simulink model "linear_controller_linear_plant_mks_sim"  (R2022b)
settings: Solver=VariableStepAuto  StartTime=0.0  StopTime=4500  FixedStep=0.5  RelTol=1e-6
undefined symbols (not defined in the file): u0, x0
libraries: mpclib x1
settings Model: Creator=Mitarbeiter  LastModifiedBy=Mitarbeiter

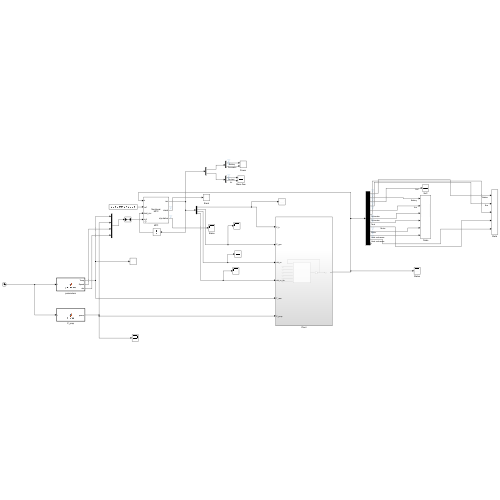
[thumbnail: Simulink's stored preview of the top-level diagram]
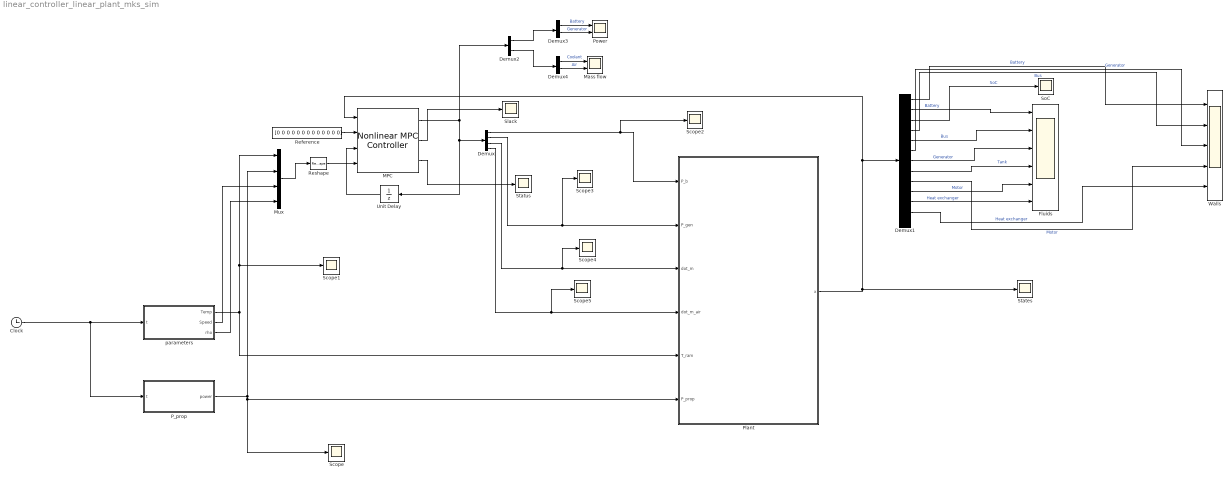
== system linear_controller_linear_plant_mks_sim ==
  Clock : Clock
  Demux : Demux
  Demux1 : Demux  Outputs=13
  Demux2 : Demux  Outputs=2
  Demux3 : Demux  Outputs=2
  Demux4 : Demux  Outputs=2
  Fluids : Scope  NumInputPorts=6
  MPC : mpclib/Nonlinear MPC Controller  nlmpcobj=nlobj  UseObjectTs=on  UseMEX=off  md_enabled=on  mvtarget_enabled=off  param_enabled=off  cost_enabled=off  mvseq_enabled=off  stateseq_enabled=off  ovseq_enabled=off  slack_enabled=on  status_enabled=on  ov_min=off  ov_max=off  mv_min=off  mv_max=off  mvrate_min=off  mvrate_max=off  state_min=off  state_max=off  ov_weight=off  mv_weight=off  mvrate_weight=off  ecr_weight=off  nlp_initialize=off
  Mass flow : Scope  NumInputPorts=2
  Mux : Mux
  P_prop : MATLAB Function  TreatAsAtomicUnit=on
  Plant : Subsystem
  Power : Scope  NumInputPorts=2
  Reference : Constant  Value=[0 0 0 0 0 0 0 0 0 0 0 0 0]  VectorParams1D=off
  Reshape : Reshape  OutputDimensionality=Row vector (2-D)
  Scope{,1..5} (6 alike) : Scope
  Slack : Scope
  SoC : Scope
  States : Scope
  Status : Scope
  Unit Delay : UnitDelay  InitialCondition=u0  SampleTime=-1  HasFrameUpgradeWarning=on
  Walls : Scope  NumInputPorts=5
  parameters : MATLAB Function  TreatAsAtomicUnit=on
  wires:
  Clock/1 -> parameters/1(t), P_prop/1(t)
  parameters/1(Temp) -> Scope1/1, Mux/1, Plant/5(T_ram)
  P_prop/1(power) -> Scope/1, Plant/6(P_prop), Mux/2
  Plant/1(x) -> MPC/1, Demux1/1, States/1
  Reference/1 -> MPC/2
  Demux/1 -> Scope2/1, Plant/1(P_b)
  Demux/2 -> Scope3/1, Plant/2(P_gen)
  MPC/1 -> Demux2/1, Demux/1, Unit Delay/1
  Mux/1 -> Reshape/1
  Unit Delay/1 -> MPC/3
  Reshape/1 -> MPC/4
  Demux1/3 -> SoC/1  "SoC"
  MPC/3 -> Status/1
  Demux/3 -> Scope4/1, Plant/3(dot_m)
  Demux/4 -> Scope5/1, Plant/4(dot_m_air)
  parameters/2(Speed) -> Mux/3
  MPC/2 -> Slack/1
  parameters/3(rho) -> Mux/4
  Demux4/1 -> Mass flow/1  "Coolant"
  Demux4/2 -> Mass flow/2  "Air"
  Demux3/2 -> Power/2  "Generator"
  Demux3/1 -> Power/1  "Battery"
  Demux2/1 -> Demux3/1
  Demux2/2 -> Demux4/1
  Demux1/1 -> Walls/1  "Battery"
  Demux1/2 -> Fluids/1  "Battery"
  Demux1/4 -> Walls/2  "Bus"
  Demux1/5 -> Fluids/2  "Bus"
  Demux1/6 -> Walls/3  "Generator"
  Demux1/7 -> Fluids/3  "Generator"
  Demux1/8 -> Fluids/4  "Tank"
  Demux1/9 -> Walls/4  "Motor"
  Demux1/10 -> Fluids/5  "Motor"
  Demux1/11 -> Fluids/6  "Heat exchanger"
  Demux1/12 -> Walls/5  "Heat exchanger"

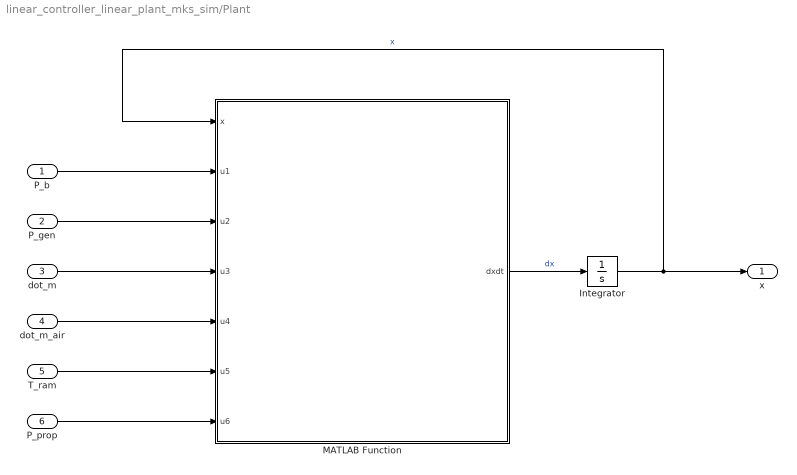
== system linear_controller_linear_plant_mks_sim/Plant ==
  P_b : Inport
  P_gen : Inport  Port=2
  dot_m : Inport  Port=3
  dot_m_air : Inport  Port=4
  T_ram : Inport  Port=5
  P_prop : Inport  Port=6
  Integrator : Integrator  InitialCondition=x0
  MATLAB Function : MATLAB Function  TreatAsAtomicUnit=on
  x : Outport
  wires:
  MATLAB Function/1(dxdt) -> Integrator/1  "dx"
  Integrator/1 -> x/1, MATLAB Function/1(x)  "x"
  P_prop/1 -> MATLAB Function/7(u6)
  P_b/1 -> MATLAB Function/2(u1)
  dot_m/1 -> MATLAB Function/4(u3)
  dot_m_air/1 -> MATLAB Function/5(u4)
  T_ram/1 -> MATLAB Function/6(u5)
  P_gen/1 -> MATLAB Function/3(u2)

== matlab function linear_controller_linear_plant_mks_sim/P_prop ==
  data: t input; power output
function power = P_prop(t)
    T_off = 60;
    t_cruise = 420;
    t_descent = 3660;
    t_landing = 4020;
    t_taxi = 4080;
    t_final = 4440;
    
    step = 636e3;
    P_slope_1 = (262e3 - 636e3)/(t_cruise - T_off);
    P_slope_2 = (114e3 - 262e3)/(t_landing - t_descent);
    P_slope_3 = (158e3 - 114e3)/(t_taxi - t_landing);
    P_slope_4 = (40e3 - 158e3)/(t_final - t_taxi);
    
    
    
    p_ramp1 = zeros(size(t));
    p_ramp1(t >= T_off) = P_slope_1 * (t(t >= T_off) - T_off);
    
    p_ramp2 = zeros(size(t));
    p_ramp2(t >= t_cruise) = -P_slope_1 * (t(t >= t_cruise) - t_cruise);
    
    p_ramp3 = zeros(size(t));
    p_ramp3(t >= t_descent) = P_slope_2 * (t(t >= t_descent) - t_descent);
    
    p_ramp4 = zeros(size(t));
    p_ramp4(t >= t_landing) = (P_slope_3 - P_slope_2) * (t(t >= t_landing) - t_landing);
    
    p_ramp5 = zeros(size(t));
    p_ramp5(t >= t_taxi) = (P_slope_4 - P_slope_3) * (t(t >= t_taxi) - t_taxi);
    
    power = step + p_ramp1 + p_ramp2 + p_ramp3 + p_ramp4 + p_ramp5;
    power(power < 0) = 0;
end

== matlab function linear_controller_linear_plant_mks_sim/Plant/MATLAB Function ==
  data: x input; dxdt output; u1 input; u2 input; u3 input; u4 input; u5 input; u6 input
function dxdt = fcn(x,u1,u2,u3,u4,u5,u6)

 dxdt = aircraft_dynamics_linear(x,[u1;u2;u3;u4;u5;u6]);

== matlab function linear_controller_linear_plant_mks_sim/parameters ==
  data: t input; Temp output; Speed output; rho output
function [Temp, Speed, rho] = parameters(t)
    %% Calculates aircraft altitude in ft and m

    T_off = 60;
    t_cruise = 420;
    t_landing = 3660;
    t_final = 4440;

    r_slope = (4000-50)/(t_cruise-T_off);
    r_slope2 =(0-4000)/(t_final-t_landing);
    
    step = 50;
    
    r_ramp1 = zeros(size(t));
    r_ramp1(t >= T_off) = r_slope * (t(t >= T_off) - T_off);
    
    r_ramp2 = zeros(size(t));
    r_ramp2(t >= t_cruise) = -r_slope * (t(t >= t_cruise) - t_cruise);
    
    r_ramp3 = zeros(size(t));
    r_ramp3(t >= t_landing) = r_slope2 * (t(t >= t_landing) - t_landing);
    
    h = step + r_ramp1 + r_ramp2 + r_ramp3;
    h(h < 0) = 0;
    
    h = 0.3048 * h;   % convert from feet to meters

    %% Calculates the ambient temperature and speed of sound (Obtained from Bing AI)
    Gamma = 1.4; % air specific heat ratio
    R = 287.053; % J/(kg.K) % gas constant
    T_amp = -6.5 * 1e-3 * h + 15;  % ambient temperature
    a = sqrt(Gamma * R * (T_amp + 273.15)); % speed of sound

    %% Calculates aircraft speed in knots; converted to Mach and m/s

    s_slope_1 = 77/60; %0.25 / 1
    s_slope_2 = (125 - 77) / (t_cruise - T_off);
    s_slope_3 = (78 - 125) / (t_final - t_landing);
    
    S_ramp = zeros(size(t));
    S_ramp(t <= T_off) = s_slope_1 * t(t <= T_off);
    
    S_ramp1 = zeros(size(t));
    S_ramp1(t > T_off & t < t_cruise) = s_slope_2 * (t(t > T_off & t < t_cruise) - T_off) + 77;
    
    S_ramp2 = zeros(size(t));
    S_ramp2(t >= t_cruise & t <= t_landing) = 125;
    
    S_ramp3 = zeros(size(t));
    S_ramp3(t > t_landing & t <= t_final) = s_slope_3 * (t(t > t_landing & t <= t_final) - t_landing) + 125;
    
    S_ramp4 = zeros(size(t));
    S_ramp4(t > t_final) = s_slope_3 * (t(t > t_final) - t_final) + 78;
    
    
    knot = S_ramp + S_ramp1 + S_ramp2 + S_ramp3 + S_ramp4; % True aircraft speed (TSA) in knots
    
    knot = 0.5144 * knot; %  TSA in m/s 
    Mach = knot / a; % Mach number

    Speed = Mach * 343; % Convert Mach to m/s
    %% Calculates the ram temperature
    Temp = T_amp * (1+Mach^2 * ((Gamma-1)/2));

    %% Calculate Pressure altitude and air density

    P0 = 101325; % Pressure at standard see level in Pascal
    P = P0 * (1 - 2.25577e-5 * h).^5.25588; % Pressure altitude % Obtained from Bing AI

    rho = P/(R* (T_amp+273.15));
end
